simulink model "observador_KM"  (R2021a)
settings: Solver=ode4  StartTime=0.0  StopTime=20  FixedStep=0.001  RelTol=1e-3
settings Model: Creator=DELL  LastModifiedBy=DELL

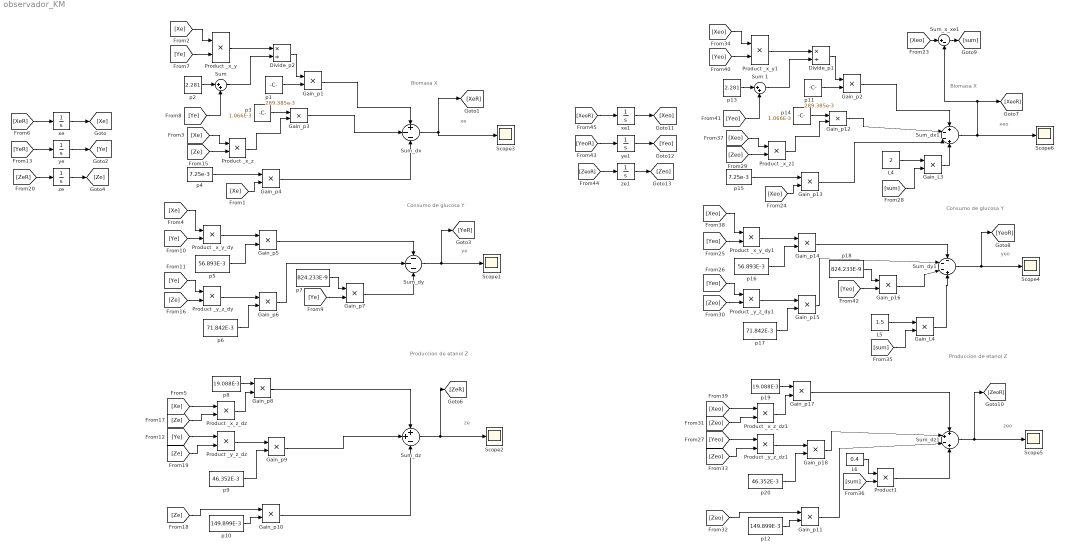
== system observador_KM ==
  note: ze
  note: ye
  note: xe
  note: Biomasa X
  note: Consumo de glucosa Y
  note: Produccion de etanol Z
  note: xeo
  note: Consumo de glucosa Y
  note: Biomasa X
  note: yeo
  note: Produccion de etanol Z
  note: zeo
  Divide_p1 : Product  Inputs=*/
  Divide_p2 : Product  Inputs=*/
  Gain_L3 : Product
  Gain_L4 : Product
  Gain_p{1..18} (18 alike) : Product
  L4 : Constant  Value=2
  L5 : Constant  Value=1.5
  L6 : Constant  Value=0.4
  Product _x_y : Product
  Product _x_y1 : Product
  Product _x_y_dy : Product
  Product _x_y_dy1 : Product
  Product _x_z : Product
  Product _x_z1 : Product
  Product _x_z_dz : Product
  Product _x_z_dz1 : Product
  Product _y_z_dy : Product
  Product _y_z_dy1 : Product
  Product _y_z_dz : Product
  Product _y_z_dz1 : Product
  Product1 : Product
  Scope{1..6} (6 alike) : Scope
  "Sum " : Sum  Inputs=|++
  Sum 1 : Sum  Inputs=|++
  Sum_dx : Sum  Inputs=+--
  Sum_dx1 : Sum  Inputs=+--+
  Sum_dy : Sum  Inputs=---
  Sum_dy1 : Sum  Inputs=---+
  Sum_dz : Sum  Inputs=++-
  Sum_dz1 : Sum  Inputs=++-+
  Sum_x_xe1 : Sum  Inputs=|+-
  p1 : Constant  Value=289.385e-3
  p10 : Constant  Value=149.899E-3
  p11 : Constant  Value=289.385e-3
  p12 : Constant  Value=149.899E-3
  p13 : Constant  Value=2.281
  p14 : Constant  Value=1.066E-3
  p15 : Constant  Value=7.25e-3
  p16 : Constant  Value=56.893E-3
  p17 : Constant  Value=71.842E-3
  p18 : Constant  Value=824.233E-9
  p19 : Constant  Value=19.088E-3
  p2 : Constant  Value=2.281
  p20 : Constant  Value=46.352E-3
  p3 : Constant  Value=1.066E-3
  p4 : Constant  Value=7.25e-3
  p5 : Constant  Value=56.893E-3
  p6 : Constant  Value=71.842E-3
  p7 : Constant  Value=824.233E-9
  p8 : Constant  Value=19.088E-3
  p9 : Constant  Value=46.352E-3
  xe : Integrator  InitialCondition=1
  xe1 : Integrator  InitialCondition=1
  ye : Integrator  InitialCondition=21
  ye1 : Integrator  InitialCondition=21
  ze : Integrator  InitialCondition=0.1
  ze1 : Integrator  InitialCondition=0.1
  wires:
  Sum_dx/1 -> [XeR], Scope3/1
  Sum_dy/1 -> [YeR], Scope1/1
  p2/1 -> "Sum "/1
  Product _x_y/1 -> Divide_p2/1
  "Sum "/1 -> Divide_p2/2
  Divide_p2/1 -> Gain_p1/1
  p1/1 -> Gain_p1/2
  p3/1 -> Gain_p3/1
  Product _x_z/1 -> Gain_p3/2
  p4/1 -> Gain_p4/1
  Gain_p1/1 -> Sum_dx/1
  Gain_p3/1 -> Sum_dx/2
  Gain_p4/1 -> Sum_dx/3
  Product _x_y_dy/1 -> Gain_p5/1
  p5/1 -> Gain_p5/2
  Product _y_z_dy/1 -> Gain_p6/1
  p6/1 -> Gain_p6/2
  p7/1 -> Gain_p7/1
  Gain_p5/1 -> Sum_dy/1
  Gain_p6/1 -> Sum_dy/2
  Gain_p7/1 -> Sum_dy/3
  p8/1 -> Gain_p8/1
  Product _x_z_dz/1 -> Gain_p8/2
  Product _y_z_dz/1 -> Gain_p9/1
  p9/1 -> Gain_p9/2
  p10/1 -> Gain_p10/2
  Gain_p8/1 -> Sum_dz/1
  Gain_p9/1 -> Sum_dz/2
  Gain_p10/1 -> Sum_dz/3
  Sum_dz/1 -> [ZeR], Scope2/1
  xe/1 -> [Xe]
  [Xe] -> Gain_p4/2
  [Xe] -> Product _x_y/1
  [Xe] -> Product _x_z/1
  [Xe] -> Product _x_y_dy/1
  [Xe] -> Product _x_z_dz/1
  [XeR] -> xe/1
  ye/1 -> [Ye]
  [Ye] -> Product _x_y/2
  [Ye] -> "Sum "/2
  [Ye] -> Gain_p7/2
  [Ye] -> Product _x_y_dy/2
  [Ye] -> Product _y_z_dy/1
  [Ye] -> Product _y_z_dz/1
  [YeR] -> ye/1
  ze/1 -> [Ze]
  [Ze] -> Product _x_z/2
  [Ze] -> Product _y_z_dy/2
  [Ze] -> Product _x_z_dz/2
  [Ze] -> Gain_p10/1
  [Ze] -> Product _y_z_dz/2
  [ZeR] -> ze/1
  [sum] -> Product1/2
  [sum] -> Gain_L3/2
  [Yeo] -> Product _x_y_dy1/2
  [Yeo] -> Gain_p16/2
  [Zeo] -> Product _x_z1/2
  [Xeo] -> Product _x_z_dz1/1
  [Xeo] -> Product _x_z1/1
  [Yeo] -> Product _y_z_dy1/1
  [Zeo] -> Product _x_z_dz1/2
  [Yeo] -> Sum 1/2
  Gain_p13/1 -> Sum_dx1/3
  Gain_p17/1 -> Sum_dz1/1
  Product _x_y1/1 -> Divide_p1/1
  p13/1 -> Sum 1/1
  Gain_p16/1 -> Sum_dy1/3
  [Xeo] -> Sum_x_xe1/1
  [Zeo] -> Product _y_z_dy1/2
  Gain_p18/1 -> Sum_dz1/2
  Divide_p1/1 -> Gain_p2/1
  Gain_p12/1 -> Sum_dx1/2
  [Yeo] -> Product _x_y1/2
  Sum_x_xe1/1 -> [sum]
  Gain_p15/1 -> Sum_dy1/2
  L5/1 -> Gain_L4/1
  L4/1 -> Gain_L3/1
  Gain_p11/1 -> Sum_dz1/3
  p17/1 -> Gain_p15/2
  Product _y_z_dy1/1 -> Gain_p15/1
  [Xeo] -> Product _x_y1/1
  p12/1 -> Gain_p11/2
  [sum] -> Gain_L4/2
  p11/1 -> Gain_p2/2
  Product _x_z_dz1/1 -> Gain_p17/2
  Sum_dx1/1 -> Scope6/1, Sum_x_xe1/2, [XeoR]
  p20/1 -> Gain_p18/2
  Product _y_z_dz1/1 -> Gain_p18/1
  Product1/1 -> Sum_dz1/4
  Gain_p14/1 -> Sum_dy1/1
  p19/1 -> Gain_p17/1
  [Yeo] -> Product _y_z_dz1/1
  Gain_L4/1 -> Sum_dy1/4
  [Zeo] -> Gain_p11/1
  Sum 1/1 -> Divide_p1/2
  Gain_L3/1 -> Sum_dx1/4
  Sum_dz1/1 -> [ZeoR], Scope5/1
  [Zeo] -> Product _y_z_dz1/2
  p14/1 -> Gain_p12/1
  [Xeo] -> Gain_p13/2
  p16/1 -> Gain_p14/2
  Product _x_y_dy1/1 -> Gain_p14/1
  p15/1 -> Gain_p13/1
  p18/1 -> Gain_p16/1
  Product _x_z1/1 -> Gain_p12/2
  Gain_p2/1 -> Sum_dx1/1
  [Xeo] -> Product _x_y_dy1/1
  L6/1 -> Product1/1
  Sum_dy1/1 -> [YeoR], Scope4/1
  [YeoR] -> ye1/1
  [XeoR] -> xe1/1
  ze1/1 -> [Zeo]
  [ZeoR] -> ze1/1
  xe1/1 -> [Xeo]
  ye1/1 -> [Yeo]
